simulink model "sim_6a"  (R2022b)
settings: Solver=FixedStepAuto  StartTime=0.0  StopTime=100  FixedStep=0.05  RelTol=1e-3
values from neighbouring files (symbols this model uses):
  a1 = 1.0125    [identa2.m]    (also in params.m)
  b1 = 0.3862    [identa2.m]    (also in params.m)
  b2 = 1.4276    [identa2.m]    (also in params.m)
settings Model: Creator=DFUNDO  LastModifiedBy=DFUNDO

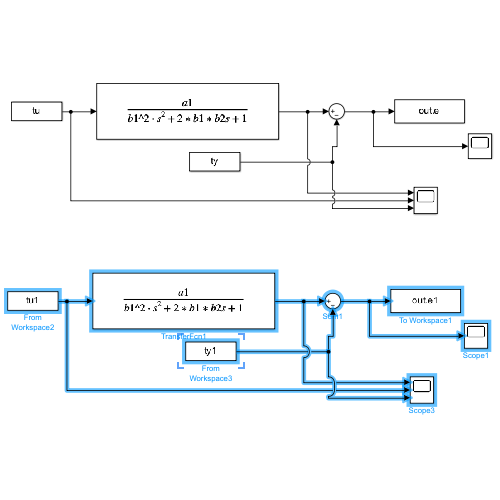
[thumbnail: Simulink's stored preview of the top-level diagram]
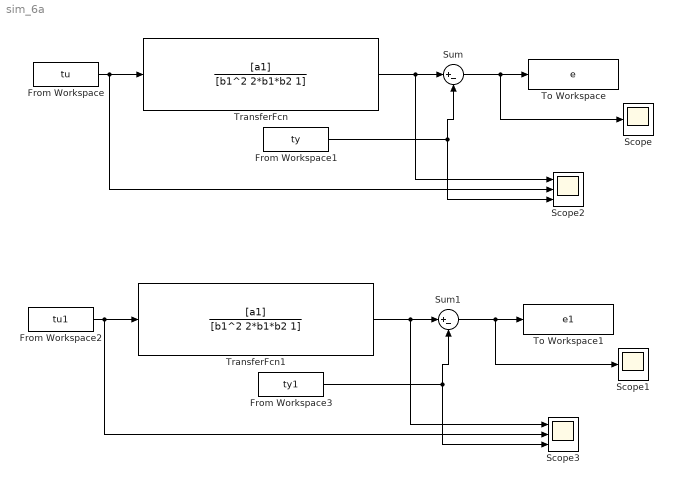
== system sim_6a ==
  From Workspace : FromWorkspace  VariableName=tu
  From Workspace1 : FromWorkspace  VariableName=ty
  From Workspace2 : FromWorkspace  VariableName=tu1
  From Workspace3 : FromWorkspace  VariableName=ty1
  Scope : Scope
  Scope1 : Scope
  Scope2 : Scope  NumInputPorts=3
  Scope3 : Scope  NumInputPorts=3
  Sum : Sum  Inputs=|+-
  Sum1 : Sum  Inputs=|+-
  To Workspace : ToWorkspace  VariableName=e  SampleTime=-1
      settings: Save2DSignal=2-D array (concatenate along first dimension)
  To Workspace1 : ToWorkspace  VariableName=e1  SampleTime=-1
      settings: Save2DSignal=2-D array (concatenate along first dimension)
  TransferFcn : TransferFcn  Numerator=[a1]  Denominator=[b1^2 2*b1*b2 1]
  TransferFcn1 : TransferFcn  Numerator=[a1]  Denominator=[b1^2 2*b1*b2 1]
  wires:
  From Workspace/1 -> TransferFcn/1, Scope2/2
  TransferFcn/1 -> Scope2/1, Sum/1
  From Workspace1/1 -> Sum/2, Scope2/3
  Sum/1 -> Scope/1, To Workspace/1
  TransferFcn1/1 -> Scope3/1, Sum1/1
  From Workspace3/1 -> Sum1/2, Scope3/3
  Sum1/1 -> Scope1/1, To Workspace1/1
  From Workspace2/1 -> TransferFcn1/1, Scope3/2
